simulink model "sampleModel7293_pp_1_1"  (R2018a)
settings: Solver=VariableStepAuto  StartTime=0.0  StopTime=10.0  RelTol=1e-3
undefined symbols (not defined in the file): DiscIntNeverNeededParam
libraries: simulink x367
(part 3 of 9)

== system sampleModel7293_pp_1_1/cfblk183 ==
  cfblk1 : Inport
  cfblk10 : Inport  Port=2
  cfblk11 : Inport  Port=3
  Action Port : ActionPort  ActionType=else
  cfblk15 : Delay
  cfblk3 : Delay  ShowEnablePort=on
      settings: InputPortMap=u0,e6
  cfblk4 : DiscreteFilter
  cfblk5 : DiscreteStateSpace  SampleTime=-1
  cfblk6 : DiscreteStateSpace  SampleTime=-1
  cfblk7 : Delay
  cfblk8 : DiscreteStateSpace  SampleTime=-1
  cfblk9 : simulink/Continuous/PID Controller  Controller=PID  TimeDomain=Discrete-time  SampleTime=-1  IntegratorMethod=Forward Euler  FilterMethod=Forward Euler  Form=Parallel  UseFilter=on  ControllerParametersSource=internal  P=1  I=1  D=0  N=100  InitialConditionSource=internal  InitialConditionForIntegrator=0  InitialConditionForFilter=0  ExternalReset=none  LimitOutput=off  UpperSaturationLimit=inf  LowerSaturationLimit=-inf  LinearizeAsGain=off  AntiWindupMode=none  Kb=1  TrackingMode=off  Kt=1  PParamMin=[]  PParamMax=[]  IParamMin=[]  IParamMax=[]  DParamMin=[]  DParamMax=[]  NParamMin=[]  NParamMax=[]  KbParamMin=[]  KbParamMax=[]  KtParamMin=[]  KtParamMax=[]  POutMin=[]  POutMax=[]  IOutMin=[]  IOutMax=[]  DOutMin=[]  DOutMax=[]  NOutMin=[]  NOutMax=[]  KbOutMin=[]  KbOutMax=[]  KtOutMin=[]  KtOutMax=[]  IntegratorOutMin=[]  IntegratorOutMax=[]  FilterOutMin=[]  FilterOutMax=[]  SumOutMin=[]  SumOutMax=[]  SumI1OutMin=[]  SumI1OutMax=[]  SumI2OutMin=[]  SumI2OutMax=[]  SumI3OutMin=[]  SumI3OutMax=[]  SumDOutMin=[]  SumDOutMax=[]  SaturationOutMin=[]  SaturationOutMax=[]  IntegratorContinuousStateAttributes=''  IntegratorStateMustResolveToSignalObject=off  IntegratorRTWStateStorageClass=Auto  FilterContinuousStateAttributes=''  FilterStateMustResolveToSignalObject=off  FilterRTWStateStorageClass=Auto  DifferentiatorICPrevScaledInput=0  DifferentiatorOutMin=[]  DifferentiatorOutMax=[]  FilterDiffOutCoefMin=[]  FilterDiffOutCoefMax=[]  SumDenOutMin=[]  SumDenOutMax=[]  SumNumOutMin=[]  SumNumOutMax=[]  ReciprocalOutMin=[]  ReciprocalOutMax=[]  DivideOutMin=[]  DivideOutMax=[]  TunerSelectOption=Transfer Function Based (PID Tuner App)
  cyemi_{518..526} (9 alike) : DataTypeConversion  OutDataTypeStr=double
  cfblk2 : Outport
  cfblk12 : Outport  Port=2
  cfblk13 : Outport  Port=3
  cfblk14 : Outport  Port=4
  wires:
  cfblk1/1 -> cfblk14/1
  cfblk4/1 -> cfblk12/1
  cfblk7/1 -> cfblk2/1, cyemi_525/1
  cfblk5/1 -> cfblk13/1, cyemi_524/1
  cyemi_518/1 -> cfblk15/1
  cfblk8/1 -> cyemi_518/1
  cyemi_519/1 -> cfblk3/1
  cfblk15/1 -> cyemi_519/1
  cyemi_520/1 -> cfblk3/2
  cfblk10/1 -> cyemi_520/1
  cyemi_521/1 -> cfblk4/1
  cfblk6/1 -> cyemi_521/1
  cyemi_522/1 -> cfblk5/1
  cfblk9/1 -> cyemi_522/1
  cyemi_523/1 -> cfblk6/1
  cfblk11/1 -> cyemi_523/1
  cyemi_524/1 -> cfblk7/1
  cyemi_525/1 -> cfblk8/1
  cyemi_526/1 -> cfblk9/1
  cfblk3/1 -> cyemi_526/1

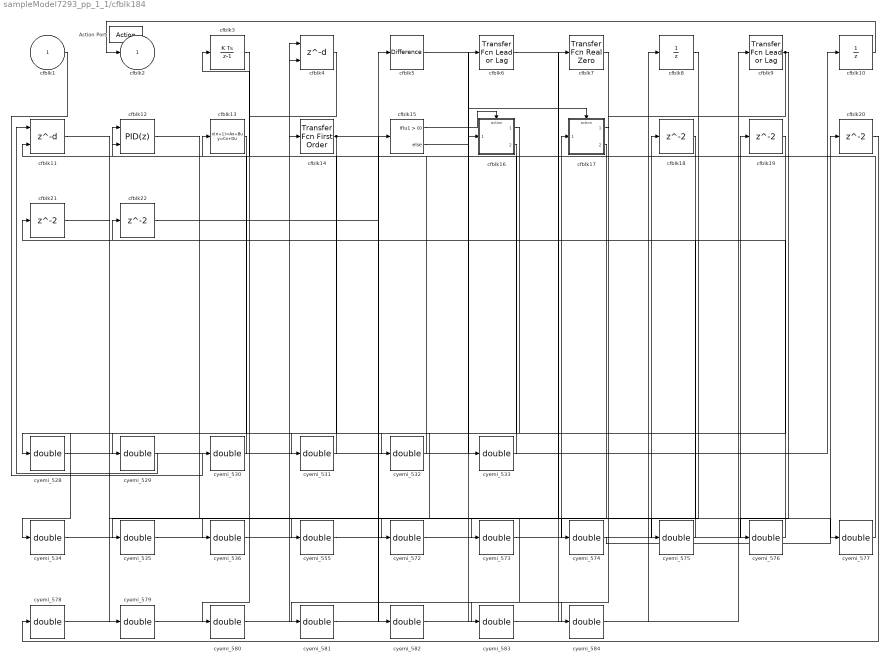
== system sampleModel7293_pp_1_1/cfblk184 ==
  cfblk1 : Inport
  Action Port : ActionPort  ActionType=then
  cfblk10 : UnitDelay  SampleTime=-1
  cfblk11 : Delay  DelayLengthSource=Input port
      settings: InputPortMap=u0,p1
  cfblk12 : simulink/Continuous/PID Controller (2DOF)  Controller=PID  TimeDomain=Discrete-time  SampleTime=-1  IntegratorMethod=Forward Euler  FilterMethod=Forward Euler  Form=Parallel  UseFilter=on  ControllerParametersSource=internal  P=1  I=1  D=0  N=100  b=1  c=1  InitialConditionSource=internal  InitialConditionForIntegrator=0  InitialConditionForFilter=0  ExternalReset=none  LimitOutput=off  UpperSaturationLimit=inf  LowerSaturationLimit=-inf  LinearizeAsGain=off  AntiWindupMode=none  Kb=1  TrackingMode=off  Kt=1  PParamMin=[]  PParamMax=[]  IParamMin=[]  IParamMax=[]  DParamMin=[]  DParamMax=[]  NParamMin=[]  NParamMax=[]  bParamMin=[]  bParamMax=[]  cParamMin=[]  cParamMax=[]  KbParamMin=[]  KbParamMax=[]  KtParamMin=[]  KtParamMax=[]  POutMin=[]  POutMax=[]  IOutMin=[]  IOutMax=[]  DOutMin=[]  DOutMax=[]  NOutMin=[]  NOutMax=[]  bOutMin=[]  bOutMax=[]  cOutMin=[]  cOutMax=[]  KbOutMin=[]  KbOutMax=[]  KtOutMin=[]  KtOutMax=[]  IntegratorOutMin=[]  IntegratorOutMax=[]  FilterOutMin=[]  FilterOutMax=[]  SumOutMin=[]  SumOutMax=[]  Sum1OutMin=[]  Sum1OutMax=[]  Sum2OutMin=[]  Sum2OutMax=[]  Sum3OutMin=[]  Sum3OutMax=[]  SumI1OutMin=[]  SumI1OutMax=[]  SumI2OutMin=[]  SumI2OutMax=[]  SumI3OutMin=[]  SumI3OutMax=[]  SumDOutMin=[]  SumDOutMax=[]  SaturationOutMin=[]  SaturationOutMax=[]  IntegratorContinuousStateAttributes=''  IntegratorStateMustResolveToSignalObject=off  IntegratorRTWStateStorageClass=Auto  FilterContinuousStateAttributes=''  FilterStateMustResolveToSignalObject=off  FilterRTWStateStorageClass=Auto  DifferentiatorICPrevScaledInput=0  DifferentiatorOutMin=[]  DifferentiatorOutMax=[]  FilterDiffOutCoefMin=[]  FilterDiffOutCoefMax=[]  SumDenOutMin=[]  SumDenOutMax=[]  SumNumOutMin=[]  SumNumOutMax=[]  ReciprocalOutMin=[]  ReciprocalOutMax=[]  DivideOutMin=[]  DivideOutMax=[]  TunerSelectOption=Transfer Function Based (PID Tuner App)
  cfblk13 : DiscreteStateSpace  SampleTime=-1
  cfblk14 : simulink/Discrete/Transfer Fcn First Order  PoleZ=0.95  ICPrevOutput=0.0  DoSatur=off
      settings: SourceProductName=Simulink
  cfblk15 : If  SampleTime=1
  cfblk16 : Subsystem  TreatAsAtomicUnit=on
  cfblk17 : Subsystem  TreatAsAtomicUnit=on
  cfblk{18..22} (5 alike) : Delay
  cfblk3 : DiscreteIntegrator  SampleTime=-1  OutDataTypeStr=double  ICPrevOutput=DiscIntNeverNeededParam  ICPrevScaledInput=DiscIntNeverNeededParam
  cfblk4 : Delay  DelayLengthSource=Input port
      settings: InputPortMap=u0,p1
  cfblk5 : simulink/Discrete/Difference  ICPrevInput=0.0  OutMin=[]  OutMax=[]  OutDataTypeStr=double  OutputDataTypeScalingMode=double  OutDataType=fixdt(1, 16)  OutScaling=2^-10  DoSatur=off
  cfblk6 : simulink/Discrete/Transfer Fcn Lead or Lag  PoleZ=0.95  ZeroZ=0.75  ICPrevOutput=0.0  ICPrevInput=0.0  DoSatur=off
      settings: SourceProductName=Simulink  SourceProductBaseCode=SL
  cfblk7 : simulink/Discrete/Transfer Fcn Real Zero  ZeroZ=0.75  ICPrevInput=0.0  DoSatur=off
      settings: SourceProductName=Simulink  SourceProductBaseCode=SL
  cfblk8 : UnitDelay  SampleTime=-1
  cfblk9 : simulink/Discrete/Transfer Fcn Lead or Lag  PoleZ=0.95  ZeroZ=0.75  ICPrevOutput=0.0  ICPrevInput=0.0  DoSatur=off
      settings: SourceProductName=Simulink  SourceProductBaseCode=SL
  cyemi_{528..536,555,572..584} (23 alike) : DataTypeConversion  OutDataTypeStr=double
  cfblk2 : Outport
  wires:
  cfblk14/1 -> cyemi_531/1, cyemi_573/1
  cfblk9/1 -> cyemi_532/1, cyemi_576/1
  cfblk10/1 -> cfblk2/1
  cfblk15/1 -> cfblk16/Action
  cfblk15/2 -> cfblk17/Action
  cyemi_528/1 -> cfblk10/1
  cfblk16/1(cfblk2) -> cyemi_528/1
  cyemi_529/1 -> cfblk11/1
  cfblk19/1 -> cyemi_529/1
  cyemi_530/1 -> cfblk11/2
  cfblk1/1 -> cyemi_530/1
  cyemi_531/1 -> cfblk12/1
  cyemi_532/1 -> cfblk12/2
  cyemi_533/1 -> cfblk13/1
  cfblk5/1 -> cyemi_533/1
  cyemi_534/1 -> cfblk14/1
  cfblk13/1 -> cyemi_534/1
  cyemi_535/1 -> cfblk15/1
  cfblk18/1 -> cyemi_535/1
  cyemi_536/1 -> cfblk16/1(cfblk1)
  cfblk4/1 -> cyemi_536/1
  cyemi_555/1 -> cfblk17/1(cfblk1)
  cfblk21/1 -> cyemi_555/1
  cyemi_572/1 -> cfblk18/1
  cfblk16/2(cfblk16) -> cyemi_572/1
  cyemi_573/1 -> cfblk19/1
  cyemi_574/1 -> cfblk20/1
  cfblk12/1 -> cyemi_574/1
  cyemi_575/1 -> cfblk21/1
  cfblk8/1 -> cyemi_575/1
  cyemi_576/1 -> cfblk22/1
  cyemi_577/1 -> cfblk3/1
  cfblk6/1 -> cyemi_577/1
  cyemi_578/1 -> cfblk4/1
  cfblk20/1 -> cyemi_578/1
  cyemi_579/1 -> cfblk4/2
  cfblk11/1 -> cyemi_579/1
  cyemi_580/1 -> cfblk5/1
  cfblk3/1 -> cyemi_580/1
  cyemi_581/1 -> cfblk6/1
  cfblk17/1(cfblk2) -> cyemi_581/1
  cyemi_582/1 -> cfblk7/1
  cfblk22/1 -> cyemi_582/1
  cyemi_583/1 -> cfblk8/1
  cfblk17/2(cfblk15) -> cyemi_583/1
  cyemi_584/1 -> cfblk9/1
  cfblk7/1 -> cyemi_584/1

== system sampleModel7293_pp_1_1/cfblk185 ==
  cfblk1 : Inport
  cfblk12 : Inport  Port=2
  cfblk13 : Inport  Port=3
  cfblk14 : Inport  Port=4
  cfblk15 : Inport  Port=5
  cfblk16 : Inport  Port=6
  Action Port : ActionPort  ActionType=else
  cfblk10 : Delay  DelayLengthSource=Input port
      settings: InputPortMap=u0,p1
  cfblk11 : If  SampleTime=1
  cfblk18 : Subsystem  TreatAsAtomicUnit=on
  cfblk19 : Subsystem  TreatAsAtomicUnit=on
  cfblk20 : Delay
  cfblk3 : simulink/Discrete/Transfer Fcn First Order  PoleZ=0.95  ICPrevOutput=0.0  DoSatur=off
      settings: SourceProductName=Simulink
  cfblk4 : simulink/Continuous/PID Controller (2DOF)  Controller=PID  TimeDomain=Discrete-time  SampleTime=-1  IntegratorMethod=Forward Euler  FilterMethod=Forward Euler  Form=Parallel  UseFilter=on  ControllerParametersSource=internal  P=1  I=1  D=0  N=100  b=1  c=1  InitialConditionSource=internal  InitialConditionForIntegrator=0  InitialConditionForFilter=0  ExternalReset=none  LimitOutput=off  UpperSaturationLimit=inf  LowerSaturationLimit=-inf  LinearizeAsGain=off  AntiWindupMode=none  Kb=1  TrackingMode=off  Kt=1  PParamMin=[]  PParamMax=[]  IParamMin=[]  IParamMax=[]  DParamMin=[]  DParamMax=[]  NParamMin=[]  NParamMax=[]  bParamMin=[]  bParamMax=[]  cParamMin=[]  cParamMax=[]  KbParamMin=[]  KbParamMax=[]  KtParamMin=[]  KtParamMax=[]  POutMin=[]  POutMax=[]  IOutMin=[]  IOutMax=[]  DOutMin=[]  DOutMax=[]  NOutMin=[]  NOutMax=[]  bOutMin=[]  bOutMax=[]  cOutMin=[]  cOutMax=[]  KbOutMin=[]  KbOutMax=[]  KtOutMin=[]  KtOutMax=[]  IntegratorOutMin=[]  IntegratorOutMax=[]  FilterOutMin=[]  FilterOutMax=[]  SumOutMin=[]  SumOutMax=[]  Sum1OutMin=[]  Sum1OutMax=[]  Sum2OutMin=[]  Sum2OutMax=[]  Sum3OutMin=[]  Sum3OutMax=[]  SumI1OutMin=[]  SumI1OutMax=[]  SumI2OutMin=[]  SumI2OutMax=[]  SumI3OutMin=[]  SumI3OutMax=[]  SumDOutMin=[]  SumDOutMax=[]  SaturationOutMin=[]  SaturationOutMax=[]  IntegratorContinuousStateAttributes=''  IntegratorStateMustResolveToSignalObject=off  IntegratorRTWStateStorageClass=Auto  FilterContinuousStateAttributes=''  FilterStateMustResolveToSignalObject=off  FilterRTWStateStorageClass=Auto  DifferentiatorICPrevScaledInput=0  DifferentiatorOutMin=[]  DifferentiatorOutMax=[]  FilterDiffOutCoefMin=[]  FilterDiffOutCoefMax=[]  SumDenOutMin=[]  SumDenOutMax=[]  SumNumOutMin=[]  SumNumOutMax=[]  ReciprocalOutMin=[]  ReciprocalOutMax=[]  DivideOutMin=[]  DivideOutMax=[]  TunerSelectOption=Transfer Function Based (PID Tuner App)
  cfblk5 : simulink/Discrete/Tapped Delay  vinit=0.0  samptime=-1  NumDelays=1  DelayOrder=Oldest  includeCurrent=off
  cfblk6 : simulink/Discrete/Transfer Fcn Lead or Lag  PoleZ=0.95  ZeroZ=0.75  ICPrevOutput=0.0  ICPrevInput=0.0  DoSatur=off
      settings: SourceProductName=Simulink  SourceProductBaseCode=SL
  cfblk7 : simulink/Continuous/PID Controller (2DOF)  Controller=PID  TimeDomain=Discrete-time  SampleTime=-1  IntegratorMethod=Forward Euler  FilterMethod=Forward Euler  Form=Parallel  UseFilter=on  ControllerParametersSource=internal  P=1  I=1  D=0  N=100  b=1  c=1  InitialConditionSource=internal  InitialConditionForIntegrator=0  InitialConditionForFilter=0  ExternalReset=none  LimitOutput=off  UpperSaturationLimit=inf  LowerSaturationLimit=-inf  LinearizeAsGain=off  AntiWindupMode=none  Kb=1  TrackingMode=off  Kt=1  PParamMin=[]  PParamMax=[]  IParamMin=[]  IParamMax=[]  DParamMin=[]  DParamMax=[]  NParamMin=[]  NParamMax=[]  bParamMin=[]  bParamMax=[]  cParamMin=[]  cParamMax=[]  KbParamMin=[]  KbParamMax=[]  KtParamMin=[]  KtParamMax=[]  POutMin=[]  POutMax=[]  IOutMin=[]  IOutMax=[]  DOutMin=[]  DOutMax=[]  NOutMin=[]  NOutMax=[]  bOutMin=[]  bOutMax=[]  cOutMin=[]  cOutMax=[]  KbOutMin=[]  KbOutMax=[]  KtOutMin=[]  KtOutMax=[]  IntegratorOutMin=[]  IntegratorOutMax=[]  FilterOutMin=[]  FilterOutMax=[]  SumOutMin=[]  SumOutMax=[]  Sum1OutMin=[]  Sum1OutMax=[]  Sum2OutMin=[]  Sum2OutMax=[]  Sum3OutMin=[]  Sum3OutMax=[]  SumI1OutMin=[]  SumI1OutMax=[]  SumI2OutMin=[]  SumI2OutMax=[]  SumI3OutMin=[]  SumI3OutMax=[]  SumDOutMin=[]  SumDOutMax=[]  SaturationOutMin=[]  SaturationOutMax=[]  IntegratorContinuousStateAttributes=''  IntegratorStateMustResolveToSignalObject=off  IntegratorRTWStateStorageClass=Auto  FilterContinuousStateAttributes=''  FilterStateMustResolveToSignalObject=off  FilterRTWStateStorageClass=Auto  DifferentiatorICPrevScaledInput=0  DifferentiatorOutMin=[]  DifferentiatorOutMax=[]  FilterDiffOutCoefMin=[]  FilterDiffOutCoefMax=[]  SumDenOutMin=[]  SumDenOutMax=[]  SumNumOutMin=[]  SumNumOutMax=[]  ReciprocalOutMin=[]  ReciprocalOutMax=[]  DivideOutMin=[]  DivideOutMax=[]  TunerSelectOption=Transfer Function Based (PID Tuner App)
  cfblk8 : DiscreteFilter
  cfblk9 : DiscreteTransferFcn
  cyemi_{591..595,607,616..625} (16 alike) : DataTypeConversion  OutDataTypeStr=double
  cfblk2 : Outport
  cfblk17 : Outport  Port=2
  wires:
  cfblk7/1 -> cfblk17/1
  cfblk6/1 -> cfblk2/1
  cfblk11/1 -> cfblk18/Action
  cfblk11/2 -> cfblk19/Action
  cyemi_591/1 -> cfblk10/1
  cfblk19/1(cfblk2) -> cyemi_591/1
  cyemi_592/1 -> cfblk10/2
  cfblk4/1 -> cyemi_592/1
  cyemi_593/1 -> cfblk11/1
  cfblk5/1 -> cyemi_593/1
  cyemi_594/1 -> cfblk18/1(cfblk1)
  cfblk9/1 -> cyemi_594/1
  cyemi_595/1 -> cfblk18/2(cfblk11)
  cfblk12/1 -> cyemi_595/1
  cyemi_607/1 -> cfblk19/1(cfblk1)
  cfblk18/2(cfblk12) -> cyemi_607/1
  cyemi_616/1 -> cfblk20/1
  cfblk18/1(cfblk2) -> cyemi_616/1
  cyemi_617/1 -> cfblk3/1
  cfblk20/1 -> cyemi_617/1
  cyemi_618/1 -> cfblk4/1
  cfblk16/1 -> cyemi_618/1
  cyemi_619/1 -> cfblk4/2
  cfblk13/1 -> cyemi_619/1
  cyemi_620/1 -> cfblk5/1
  cfblk8/1 -> cyemi_620/1
  cyemi_621/1 -> cfblk6/1
  cfblk15/1 -> cyemi_621/1
  cyemi_622/1 -> cfblk7/1
  cfblk1/1 -> cyemi_622/1
  cyemi_623/1 -> cfblk7/2
  cfblk10/1 -> cyemi_623/1
  cyemi_624/1 -> cfblk8/1
  cfblk14/1 -> cyemi_624/1
  cyemi_625/1 -> cfblk9/1
  cfblk3/1 -> cyemi_625/1

== system sampleModel7293_pp_1_1/cfblk186 ==
  cfblk1 : Inport
  cfblk5 : Inport  Port=2
  cfblk6 : Inport  Port=3
  cfblk7 : Inport  Port=4
  Action Port : ActionPort  ActionType=then
  cfblk3 : Delay  ShowEnablePort=on
      settings: InputPortMap=u0,e6
  cfblk4 : simulink/Discrete/Difference  ICPrevInput=0.0  OutMin=[]  OutMax=[]  OutDataTypeStr=double  OutputDataTypeScalingMode=double  OutDataType=fixdt(1, 16)  OutScaling=2^-10  DoSatur=off
  cyemi_630 : DataTypeConversion  OutDataTypeStr=double
  cyemi_631 : DataTypeConversion  OutDataTypeStr=double
  cyemi_632 : DataTypeConversion  OutDataTypeStr=double
  cfblk2 : Outport
  cfblk8 : Outport  Port=2
  wires:
  cfblk5/1 -> cfblk2/1
  cfblk7/1 -> cfblk8/1
  cyemi_630/1 -> cfblk3/1
  cfblk1/1 -> cyemi_630/1
  cyemi_631/1 -> cfblk3/2
  cfblk4/1 -> cyemi_631/1
  cyemi_632/1 -> cfblk4/1
  cfblk6/1 -> cyemi_632/1

== system sampleModel7293_pp_1_1/cfblk187 ==
  cfblk1 : Inport
  cfblk8 : Inport  Port=2
  cfblk9 : Inport  Port=3
  Action Port : ActionPort  ActionType=else
  cfblk11 : Subsystem  TreatAsAtomicUnit=on
  cfblk12 : Subsystem  TreatAsAtomicUnit=on
  cfblk13 : Delay
  cfblk14 : Delay
  cfblk15 : Delay
  cfblk3 : simulink/Continuous/PID Controller (2DOF)  Controller=PID  TimeDomain=Discrete-time  SampleTime=-1  IntegratorMethod=Forward Euler  FilterMethod=Forward Euler  Form=Parallel  UseFilter=on  ControllerParametersSource=internal  P=1  I=1  D=0  N=100  b=1  c=1  InitialConditionSource=internal  InitialConditionForIntegrator=0  InitialConditionForFilter=0  ExternalReset=none  LimitOutput=off  UpperSaturationLimit=inf  LowerSaturationLimit=-inf  LinearizeAsGain=off  AntiWindupMode=none  Kb=1  TrackingMode=off  Kt=1  PParamMin=[]  PParamMax=[]  IParamMin=[]  IParamMax=[]  DParamMin=[]  DParamMax=[]  NParamMin=[]  NParamMax=[]  bParamMin=[]  bParamMax=[]  cParamMin=[]  cParamMax=[]  KbParamMin=[]  KbParamMax=[]  KtParamMin=[]  KtParamMax=[]  POutMin=[]  POutMax=[]  IOutMin=[]  IOutMax=[]  DOutMin=[]  DOutMax=[]  NOutMin=[]  NOutMax=[]  bOutMin=[]  bOutMax=[]  cOutMin=[]  cOutMax=[]  KbOutMin=[]  KbOutMax=[]  KtOutMin=[]  KtOutMax=[]  IntegratorOutMin=[]  IntegratorOutMax=[]  FilterOutMin=[]  FilterOutMax=[]  SumOutMin=[]  SumOutMax=[]  Sum1OutMin=[]  Sum1OutMax=[]  Sum2OutMin=[]  Sum2OutMax=[]  Sum3OutMin=[]  Sum3OutMax=[]  SumI1OutMin=[]  SumI1OutMax=[]  SumI2OutMin=[]  SumI2OutMax=[]  SumI3OutMin=[]  SumI3OutMax=[]  SumDOutMin=[]  SumDOutMax=[]  SaturationOutMin=[]  SaturationOutMax=[]  IntegratorContinuousStateAttributes=''  IntegratorStateMustResolveToSignalObject=off  IntegratorRTWStateStorageClass=Auto  FilterContinuousStateAttributes=''  FilterStateMustResolveToSignalObject=off  FilterRTWStateStorageClass=Auto  DifferentiatorICPrevScaledInput=0  DifferentiatorOutMin=[]  DifferentiatorOutMax=[]  FilterDiffOutCoefMin=[]  FilterDiffOutCoefMax=[]  SumDenOutMin=[]  SumDenOutMax=[]  SumNumOutMin=[]  SumNumOutMax=[]  ReciprocalOutMin=[]  ReciprocalOutMax=[]  DivideOutMin=[]  DivideOutMax=[]  TunerSelectOption=Transfer Function Based (PID Tuner App)
  cfblk4 : simulink/Discrete/Tapped Delay  vinit=0.0  samptime=-1  NumDelays=1  DelayOrder=Oldest  includeCurrent=off
  cfblk5 : simulink/Continuous/PID Controller (2DOF)  Controller=PID  TimeDomain=Discrete-time  SampleTime=-1  IntegratorMethod=Forward Euler  FilterMethod=Forward Euler  Form=Parallel  UseFilter=on  ControllerParametersSource=internal  P=1  I=1  D=0  N=100  b=1  c=1  InitialConditionSource=internal  InitialConditionForIntegrator=0  InitialConditionForFilter=0  ExternalReset=none  LimitOutput=off  UpperSaturationLimit=inf  LowerSaturationLimit=-inf  LinearizeAsGain=off  AntiWindupMode=none  Kb=1  TrackingMode=off  Kt=1  PParamMin=[]  PParamMax=[]  IParamMin=[]  IParamMax=[]  DParamMin=[]  DParamMax=[]  NParamMin=[]  NParamMax=[]  bParamMin=[]  bParamMax=[]  cParamMin=[]  cParamMax=[]  KbParamMin=[]  KbParamMax=[]  KtParamMin=[]  KtParamMax=[]  POutMin=[]  POutMax=[]  IOutMin=[]  IOutMax=[]  DOutMin=[]  DOutMax=[]  NOutMin=[]  NOutMax=[]  bOutMin=[]  bOutMax=[]  cOutMin=[]  cOutMax=[]  KbOutMin=[]  KbOutMax=[]  KtOutMin=[]  KtOutMax=[]  IntegratorOutMin=[]  IntegratorOutMax=[]  FilterOutMin=[]  FilterOutMax=[]  SumOutMin=[]  SumOutMax=[]  Sum1OutMin=[]  Sum1OutMax=[]  Sum2OutMin=[]  Sum2OutMax=[]  Sum3OutMin=[]  Sum3OutMax=[]  SumI1OutMin=[]  SumI1OutMax=[]  SumI2OutMin=[]  SumI2OutMax=[]  SumI3OutMin=[]  SumI3OutMax=[]  SumDOutMin=[]  SumDOutMax=[]  SaturationOutMin=[]  SaturationOutMax=[]  IntegratorContinuousStateAttributes=''  IntegratorStateMustResolveToSignalObject=off  IntegratorRTWStateStorageClass=Auto  FilterContinuousStateAttributes=''  FilterStateMustResolveToSignalObject=off  FilterRTWStateStorageClass=Auto  DifferentiatorICPrevScaledInput=0  DifferentiatorOutMin=[]  DifferentiatorOutMax=[]  FilterDiffOutCoefMin=[]  FilterDiffOutCoefMax=[]  SumDenOutMin=[]  SumDenOutMax=[]  SumNumOutMin=[]  SumNumOutMax=[]  ReciprocalOutMin=[]  ReciprocalOutMax=[]  DivideOutMin=[]  DivideOutMax=[]  TunerSelectOption=Transfer Function Based (PID Tuner App)
  cfblk6 : DiscreteFilter
  cfblk7 : If  SampleTime=1
  cyemi_{636..638,651..653,660..669} (16 alike) : DataTypeConversion  OutDataTypeStr=double
  cfblk2 : Outport
  cfblk10 : Outport  Port=2
  wires:
  cfblk3/1 -> cfblk10/1
  cfblk9/1 -> cyemi_638/1, cyemi_669/1
  cfblk6/1 -> cfblk2/1, cyemi_637/1, cyemi_666/1
  cfblk12/2(cfblk10) -> cyemi_660/1, cyemi_664/1
  cfblk4/1 -> cyemi_661/1, cyemi_662/1
  cfblk7/1 -> cfblk11/Action
  cfblk7/2 -> cfblk12/Action
  cyemi_636/1 -> cfblk11/1(cfblk1)
  cfblk8/1 -> cyemi_636/1
  cyemi_637/1 -> cfblk11/2(cfblk13)
  cyemi_638/1 -> cfblk11/3(cfblk14)
  cyemi_651/1 -> cfblk12/1(cfblk1)
  cfblk5/1 -> cyemi_651/1
  cyemi_652/1 -> cfblk12/2(cfblk8)
  cfblk14/1 -> cyemi_652/1
  cyemi_653/1 -> cfblk12/3(cfblk9)
  cfblk15/1 -> cyemi_653/1
  cyemi_660/1 -> cfblk13/1
  cyemi_661/1 -> cfblk14/1
  cyemi_662/1 -> cfblk15/1
  cyemi_663/1 -> cfblk3/1
  cfblk12/1(cfblk2) -> cyemi_663/1
  cyemi_664/1 -> cfblk3/2
  cyemi_665/1 -> cfblk4/1
  cfblk11/1(cfblk2) -> cyemi_665/1
  cyemi_666/1 -> cfblk5/1
  cyemi_667/1 -> cfblk5/2
  cfblk13/1 -> cyemi_667/1
  cyemi_668/1 -> cfblk6/1
  cfblk1/1 -> cyemi_668/1
  cyemi_669/1 -> cfblk7/1

== system sampleModel7293_pp_1_1/cfblk188 ==
  cfblk1 : Inport
  cfblk9 : Inport  Port=2
  cfblk10 : Inport  Port=3
  cfblk11 : Inport  Port=4
  Action Port : ActionPort  ActionType=then
  cfblk3 : DiscreteTransferFcn
  cfblk4 : DiscreteFir
  cfblk5 : DiscreteZeroPole  Poles=[0 0.5]  Gain=1  SampleTime=-1
  cfblk6 : simulink/Discrete/Transfer Fcn First Order  PoleZ=0.95  ICPrevOutput=0.0  DoSatur=off
      settings: SourceProductName=Simulink
  cfblk7 : UnitDelay  SampleTime=-1
  cfblk8 : DiscreteIntegrator  SampleTime=-1  OutDataTypeStr=double  ICPrevOutput=DiscIntNeverNeededParam  ICPrevScaledInput=DiscIntNeverNeededParam
  cyemi_{674..679} (6 alike) : DataTypeConversion  OutDataTypeStr=double
  cfblk2 : Outport
  cfblk12 : Outport  Port=2
  wires:
  cfblk7/1 -> cfblk12/1
  cfblk4/1 -> cfblk2/1
  cyemi_674/1 -> cfblk3/1
  cfblk1/1 -> cyemi_674/1
  cyemi_675/1 -> cfblk4/1
  cfblk5/1 -> cyemi_675/1
  cyemi_676/1 -> cfblk5/1
  cfblk6/1 -> cyemi_676/1
  cyemi_677/1 -> cfblk6/1
  cfblk8/1 -> cyemi_677/1
  cyemi_678/1 -> cfblk7/1
  cfblk11/1 -> cyemi_678/1
  cyemi_679/1 -> cfblk8/1
  cfblk3/1 -> cyemi_679/1

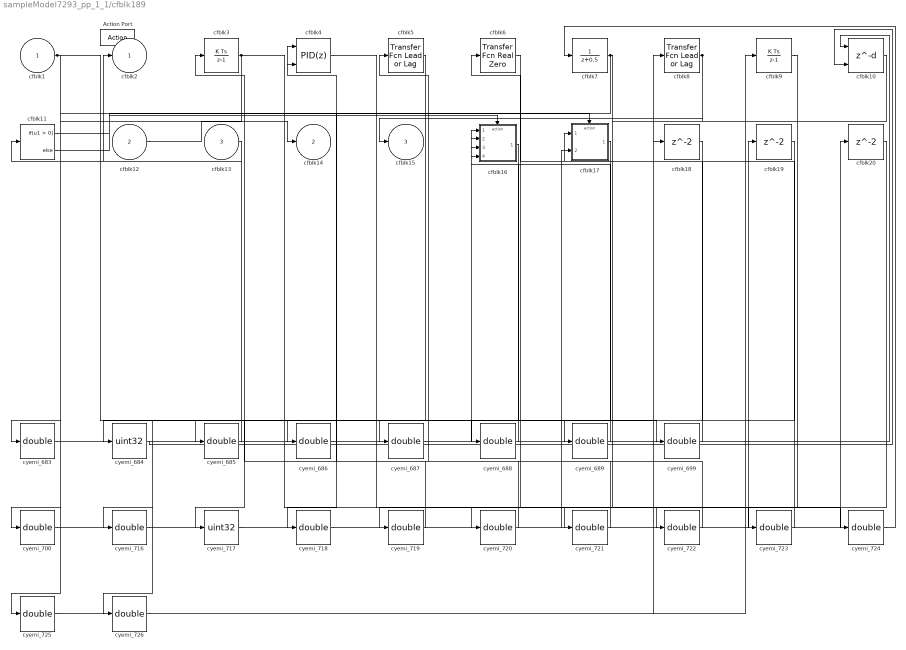
== system sampleModel7293_pp_1_1/cfblk189 ==
  cfblk1 : Inport
  cfblk12 : Inport  Port=2
  cfblk13 : Inport  Port=3
  Action Port : ActionPort  ActionType=else
  cfblk10 : Delay  DelayLengthSource=Input port
      settings: InputPortMap=u0,p1
  cfblk11 : If  SampleTime=1
  cfblk16 : Subsystem  TreatAsAtomicUnit=on
  cfblk17 : Subsystem  TreatAsAtomicUnit=on
  cfblk18 : Delay
  cfblk19 : Delay
  cfblk20 : Delay
  cfblk3 : DiscreteIntegrator  SampleTime=-1  OutDataTypeStr=double  ICPrevOutput=DiscIntNeverNeededParam  ICPrevScaledInput=DiscIntNeverNeededParam
  cfblk4 : simulink/Continuous/PID Controller (2DOF)  Controller=PID  TimeDomain=Discrete-time  SampleTime=-1  IntegratorMethod=Forward Euler  FilterMethod=Forward Euler  Form=Parallel  UseFilter=on  ControllerParametersSource=internal  P=1  I=1  D=0  N=100  b=1  c=1  InitialConditionSource=internal  InitialConditionForIntegrator=0  InitialConditionForFilter=0  ExternalReset=none  LimitOutput=off  UpperSaturationLimit=inf  LowerSaturationLimit=-inf  LinearizeAsGain=off  AntiWindupMode=none  Kb=1  TrackingMode=off  Kt=1  PParamMin=[]  PParamMax=[]  IParamMin=[]  IParamMax=[]  DParamMin=[]  DParamMax=[]  NParamMin=[]  NParamMax=[]  bParamMin=[]  bParamMax=[]  cParamMin=[]  cParamMax=[]  KbParamMin=[]  KbParamMax=[]  KtParamMin=[]  KtParamMax=[]  POutMin=[]  POutMax=[]  IOutMin=[]  IOutMax=[]  DOutMin=[]  DOutMax=[]  NOutMin=[]  NOutMax=[]  bOutMin=[]  bOutMax=[]  cOutMin=[]  cOutMax=[]  KbOutMin=[]  KbOutMax=[]  KtOutMin=[]  KtOutMax=[]  IntegratorOutMin=[]  IntegratorOutMax=[]  FilterOutMin=[]  FilterOutMax=[]  SumOutMin=[]  SumOutMax=[]  Sum1OutMin=[]  Sum1OutMax=[]  Sum2OutMin=[]  Sum2OutMax=[]  Sum3OutMin=[]  Sum3OutMax=[]  SumI1OutMin=[]  SumI1OutMax=[]  SumI2OutMin=[]  SumI2OutMax=[]  SumI3OutMin=[]  SumI3OutMax=[]  SumDOutMin=[]  SumDOutMax=[]  SaturationOutMin=[]  SaturationOutMax=[]  IntegratorContinuousStateAttributes=''  IntegratorStateMustResolveToSignalObject=off  IntegratorRTWStateStorageClass=Auto  FilterContinuousStateAttributes=''  FilterStateMustResolveToSignalObject=off  FilterRTWStateStorageClass=Auto  DifferentiatorICPrevScaledInput=0  DifferentiatorOutMin=[]  DifferentiatorOutMax=[]  FilterDiffOutCoefMin=[]  FilterDiffOutCoefMax=[]  SumDenOutMin=[]  SumDenOutMax=[]  SumNumOutMin=[]  SumNumOutMax=[]  ReciprocalOutMin=[]  ReciprocalOutMax=[]  DivideOutMin=[]  DivideOutMax=[]  TunerSelectOption=Transfer Function Based (PID Tuner App)
  cfblk5 : simulink/Discrete/Transfer Fcn Lead or Lag  PoleZ=0.95  ZeroZ=0.75  ICPrevOutput=0.0  ICPrevInput=0.0  DoSatur=off
      settings: SourceProductName=Simulink  SourceProductBaseCode=SL
  cfblk6 : simulink/Discrete/Transfer Fcn Real Zero  ZeroZ=0.75  ICPrevInput=0.0  DoSatur=off
      settings: SourceProductName=Simulink  SourceProductBaseCode=SL
  cfblk7 : DiscreteTransferFcn
  cfblk8 : simulink/Discrete/Transfer Fcn Lead or Lag  PoleZ=0.95  ZeroZ=0.75  ICPrevOutput=0.0  ICPrevInput=0.0  DoSatur=off
      settings: SourceProductName=Simulink  SourceProductBaseCode=SL
  cfblk9 : DiscreteIntegrator  SampleTime=-1  OutDataTypeStr=double  ICPrevOutput=DiscIntNeverNeededParam  ICPrevScaledInput=DiscIntNeverNeededParam
  cyemi_{683,685..689,699..700,716,718..726} (18 alike) : DataTypeConversion  OutDataTypeStr=double
  cyemi_684 : DataTypeConversion  OutDataTypeStr=uint32
  cyemi_717 : DataTypeConversion  OutDataTypeStr=uint32
  cfblk2 : Outport
  cfblk14 : Outport  Port=2
  cfblk15 : Outport  Port=3
  wires:
  cfblk1/1 -> cyemi_683/1, cyemi_687/1
  cfblk12/1 -> cfblk14/1
  cfblk7/1 -> cyemi_688/1, cyemi_718/1, cyemi_721/1, cyemi_725/1
  cfblk3/1 -> cyemi_699/1, cyemi_700/1, cyemi_724/1
  cfblk8/1 -> cfblk15/1, cyemi_689/1
  cfblk13/1 -> cfblk2/1
  cfblk11/1 -> cfblk16/Action
  cfblk11/2 -> cfblk17/Action
  cyemi_683/1 -> cfblk10/1
  cyemi_684/1 -> cfblk10/2
  cfblk19/1 -> cyemi_684/1
  cyemi_685/1 -> cfblk11/1
  cfblk10/1 -> cyemi_685/1
  cyemi_686/1 -> cfblk16/1(cfblk1)
  cfblk18/1 -> cyemi_686/1
  cyemi_687/1 -> cfblk16/2(cfblk11)
  cyemi_688/1 -> cfblk16/3(cfblk12)
  cyemi_689/1 -> cfblk16/4(cfblk13)
  cyemi_699/1 -> cfblk17/1(cfblk1)
  cyemi_700/1 -> cfblk17/2(cfblk15)
  cyemi_716/1 -> cfblk18/1
  cfblk5/1 -> cyemi_716/1
  cyemi_717/1 -> cfblk19/1
  cfblk17/1(cfblk2) -> cyemi_717/1
  cyemi_718/1 -> cfblk20/1
  cyemi_719/1 -> cfblk3/1
  cfblk20/1 -> cyemi_719/1
  cyemi_720/1 -> cfblk4/1
  cfblk6/1 -> cyemi_720/1
  cyemi_721/1 -> cfblk4/2
  cyemi_722/1 -> cfblk5/1
  cfblk4/1 -> cyemi_722/1
  cyemi_723/1 -> cfblk6/1
  cfblk9/1 -> cyemi_723/1
  cyemi_724/1 -> cfblk7/1
  cyemi_725/1 -> cfblk8/1
  cyemi_726/1 -> cfblk9/1
  cfblk16/1(cfblk2) -> cyemi_726/1

== system sampleModel7293_pp_1_1/cfblk190 ==
  cfblk1 : Inport
  Action Port : ActionPort  ActionType=then
  cfblk10 : Subsystem  TreatAsAtomicUnit=on
  cfblk11 : Delay
  cfblk12 : Delay
  cfblk13 : Delay
  cfblk3 : simulink/Discrete/Transfer Fcn Lead or Lag  PoleZ=0.95  ZeroZ=0.75  ICPrevOutput=0.0  ICPrevInput=0.0  DoSatur=off
      settings: SourceProductName=Simulink  SourceProductBaseCode=SL
  cfblk4 : UnitDelay  SampleTime=-1
  cfblk5 : simulink/Discrete/Transfer Fcn Real Zero  ZeroZ=0.75  ICPrevInput=0.0  DoSatur=off
      settings: SourceProductName=Simulink  SourceProductBaseCode=SL
  cfblk6 : If  SampleTime=1
  cfblk9 : Subsystem  TreatAsAtomicUnit=on
  cyemi_{729..730,749..756} (10 alike) : DataTypeConversion  OutDataTypeStr=double
  cfblk2 : Outport
  cfblk7 : Outport  Port=2
  cfblk8 : Outport  Port=3
  wires:
  cfblk9/1(cfblk2) -> cfblk2/1, cyemi_754/1
  cfblk10/2(cfblk15) -> cfblk7/1, cyemi_753/1
  cfblk4/1 -> cfblk8/1, cyemi_751/1
  cfblk6/1 -> cfblk9/Action
  cfblk6/2 -> cfblk10/Action
  cyemi_729/1 -> cfblk10/1(cfblk1)
  cfblk11/1 -> cyemi_729/1
  cyemi_730/1 -> cfblk10/2(cfblk14)
  cfblk1/1 -> cyemi_730/1
  cyemi_749/1 -> cfblk11/1
  cfblk3/1 -> cyemi_749/1
  cyemi_750/1 -> cfblk12/1
  cfblk10/1(cfblk2) -> cyemi_750/1
  cyemi_751/1 -> cfblk13/1
  cyemi_752/1 -> cfblk3/1
  cfblk5/1 -> cyemi_752/1
  cyemi_753/1 -> cfblk4/1
  cyemi_754/1 -> cfblk5/1
  cyemi_755/1 -> cfblk6/1
  cfblk12/1 -> cyemi_755/1
  cyemi_756/1 -> cfblk9/1(cfblk1)
  cfblk13/1 -> cyemi_756/1

== system sampleModel7293_pp_1_1/cfblk191 ==
  cfblk1 : Inport
  cfblk8 : Inport  Port=2
  Action Port : ActionPort  ActionType=else
  cfblk10 : Delay
  cfblk3 : DiscreteFir
  cfblk4 : simulink/Continuous/PID Controller (2DOF)  Controller=PID  TimeDomain=Discrete-time  SampleTime=-1  IntegratorMethod=Forward Euler  FilterMethod=Forward Euler  Form=Parallel  UseFilter=on  ControllerParametersSource=internal  P=1  I=1  D=0  N=100  b=1  c=1  InitialConditionSource=internal  InitialConditionForIntegrator=0  InitialConditionForFilter=0  ExternalReset=none  LimitOutput=off  UpperSaturationLimit=inf  LowerSaturationLimit=-inf  LinearizeAsGain=off  AntiWindupMode=none  Kb=1  TrackingMode=off  Kt=1  PParamMin=[]  PParamMax=[]  IParamMin=[]  IParamMax=[]  DParamMin=[]  DParamMax=[]  NParamMin=[]  NParamMax=[]  bParamMin=[]  bParamMax=[]  cParamMin=[]  cParamMax=[]  KbParamMin=[]  KbParamMax=[]  KtParamMin=[]  KtParamMax=[]  POutMin=[]  POutMax=[]  IOutMin=[]  IOutMax=[]  DOutMin=[]  DOutMax=[]  NOutMin=[]  NOutMax=[]  bOutMin=[]  bOutMax=[]  cOutMin=[]  cOutMax=[]  KbOutMin=[]  KbOutMax=[]  KtOutMin=[]  KtOutMax=[]  IntegratorOutMin=[]  IntegratorOutMax=[]  FilterOutMin=[]  FilterOutMax=[]  SumOutMin=[]  SumOutMax=[]  Sum1OutMin=[]  Sum1OutMax=[]  Sum2OutMin=[]  Sum2OutMax=[]  Sum3OutMin=[]  Sum3OutMax=[]  SumI1OutMin=[]  SumI1OutMax=[]  SumI2OutMin=[]  SumI2OutMax=[]  SumI3OutMin=[]  SumI3OutMax=[]  SumDOutMin=[]  SumDOutMax=[]  SaturationOutMin=[]  SaturationOutMax=[]  IntegratorContinuousStateAttributes=''  IntegratorStateMustResolveToSignalObject=off  IntegratorRTWStateStorageClass=Auto  FilterContinuousStateAttributes=''  FilterStateMustResolveToSignalObject=off  FilterRTWStateStorageClass=Auto  DifferentiatorICPrevScaledInput=0  DifferentiatorOutMin=[]  DifferentiatorOutMax=[]  FilterDiffOutCoefMin=[]  FilterDiffOutCoefMax=[]  SumDenOutMin=[]  SumDenOutMax=[]  SumNumOutMin=[]  SumNumOutMax=[]  ReciprocalOutMin=[]  ReciprocalOutMax=[]  DivideOutMin=[]  DivideOutMax=[]  TunerSelectOption=Transfer Function Based (PID Tuner App)
  cfblk5 : simulink/Discrete/Transfer Fcn Real Zero  ZeroZ=0.75  ICPrevInput=0.0  DoSatur=off
      settings: SourceProductName=Simulink  SourceProductBaseCode=SL
  cfblk6 : Delay  DelayLengthSource=Input port
      settings: InputPortMap=u0,p1
  cfblk7 : DiscreteStateSpace  SampleTime=-1
  cfblk9 : Delay
  cyemi_{772..780} (9 alike) : DataTypeConversion  OutDataTypeStr=double
  cfblk2 : Outport
  wires:
  cfblk8/1 -> cfblk2/1
  cfblk6/1 -> cyemi_773/1, cyemi_780/1
  cyemi_772/1 -> cfblk10/1
  cfblk3/1 -> cyemi_772/1
  cyemi_773/1 -> cfblk3/1
  cyemi_774/1 -> cfblk4/1
  cfblk7/1 -> cyemi_774/1
  cyemi_775/1 -> cfblk4/2
  cfblk9/1 -> cyemi_775/1
  cyemi_776/1 -> cfblk5/1
  cfblk1/1 -> cyemi_776/1
  cyemi_777/1 -> cfblk6/1
  cfblk4/1 -> cyemi_777/1
  cyemi_778/1 -> cfblk6/2
  cfblk10/1 -> cyemi_778/1
  cyemi_779/1 -> cfblk7/1
  cfblk5/1 -> cyemi_779/1
  cyemi_780/1 -> cfblk9/1

== system sampleModel7293_pp_1_1/cfblk192 ==
  cfblk1 : Inport
  cfblk9 : Inport  Port=2
  cfblk10 : Inport  Port=3
  Action Port : ActionPort  ActionType=then
  cfblk3 : DiscreteTransferFcn
  cfblk4 : simulink/Discrete/Tapped Delay  vinit=0.0  samptime=-1  NumDelays=1  DelayOrder=Oldest  includeCurrent=off
  cfblk5 : DiscreteFir
  cfblk6 : Delay  DelayLengthSource=Input port
      settings: InputPortMap=u0,p1
  cfblk7 : simulink/Discrete/Difference  ICPrevInput=0.0  OutMin=[]  OutMax=[]  OutDataTypeStr=double  OutputDataTypeScalingMode=double  OutDataType=fixdt(1, 16)  OutScaling=2^-10  DoSatur=off
  cfblk8 : DiscreteTransferFcn
  cyemi_{784..790} (7 alike) : DataTypeConversion  OutDataTypeStr=double
  cfblk2 : Outport
  cfblk11 : Outport  Port=2
  wires:
  cfblk10/1 -> cfblk2/1
  cfblk5/1 -> cfblk11/1
  cyemi_784/1 -> cfblk3/1
  cfblk6/1 -> cyemi_784/1
  cyemi_785/1 -> cfblk4/1
  cfblk8/1 -> cyemi_785/1
  cyemi_786/1 -> cfblk5/1
  cfblk7/1 -> cyemi_786/1
  cyemi_787/1 -> cfblk6/1
  cfblk1/1 -> cyemi_787/1
  cyemi_788/1 -> cfblk6/2
  cfblk4/1 -> cyemi_788/1
  cyemi_789/1 -> cfblk7/1
  cfblk3/1 -> cyemi_789/1
  cyemi_790/1 -> cfblk8/1
  cfblk9/1 -> cyemi_790/1

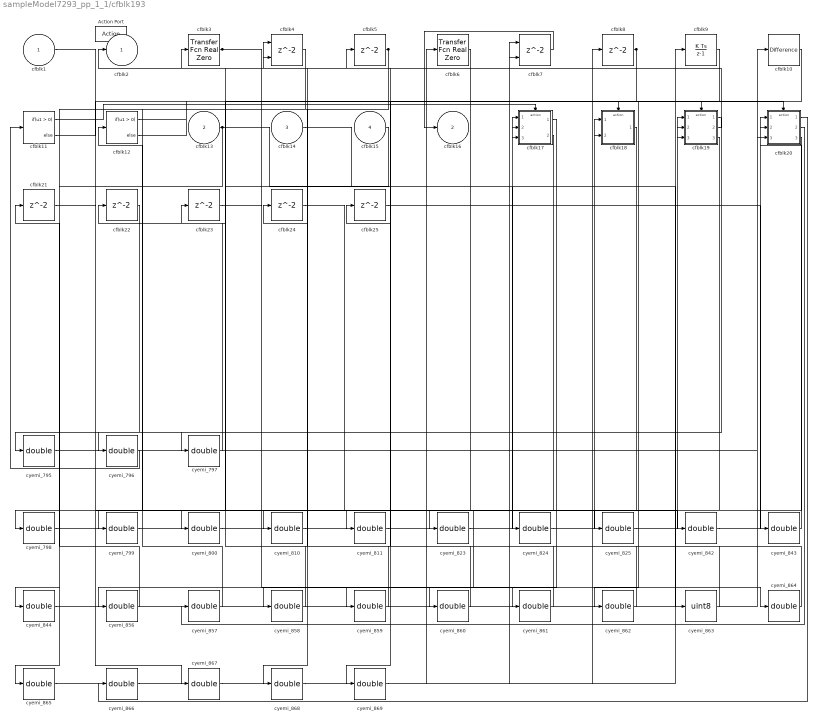
== system sampleModel7293_pp_1_1/cfblk193 ==
  cfblk1 : Inport
  cfblk13 : Inport  Port=2
  cfblk14 : Inport  Port=3
  cfblk15 : Inport  Port=4
  Action Port : ActionPort  ActionType=else
  cfblk10 : simulink/Discrete/Difference  ICPrevInput=0.0  OutMin=[]  OutMax=[]  OutDataTypeStr=double  OutputDataTypeScalingMode=double  OutDataType=fixdt(1, 16)  OutScaling=2^-10  DoSatur=off
  cfblk11 : If  SampleTime=1
  cfblk12 : If  SampleTime=1
  cfblk17 : Subsystem  TreatAsAtomicUnit=on
  cfblk18 : Subsystem  TreatAsAtomicUnit=on
  cfblk19 : Subsystem  TreatAsAtomicUnit=on
  cfblk20 : Subsystem  TreatAsAtomicUnit=on
  cfblk{5,8,21..25} (7 alike) : Delay
  cfblk3 : simulink/Discrete/Transfer Fcn Real Zero  ZeroZ=0.75  ICPrevInput=0.0  DoSatur=off
      settings: SourceProductName=Simulink  SourceProductBaseCode=SL
  cfblk4 : Delay  ShowEnablePort=on
      settings: InputPortMap=u0,e6
  cfblk6 : simulink/Discrete/Transfer Fcn Real Zero  ZeroZ=0.75  ICPrevInput=0.0  DoSatur=off
      settings: SourceProductName=Simulink  SourceProductBaseCode=SL
  cfblk7 : Delay  ShowEnablePort=on
      settings: InputPortMap=u0,e6
  cfblk9 : DiscreteIntegrator  SampleTime=-1  OutDataTypeStr=double  ICPrevOutput=DiscIntNeverNeededParam  ICPrevScaledInput=DiscIntNeverNeededParam
  cyemi_{795..800,810..811,823..825,842..844,856..862,864..869} (27 alike) : DataTypeConversion  OutDataTypeStr=double
  cyemi_863 : DataTypeConversion  OutDataTypeStr=uint8
  cfblk2 : Outport
  cfblk16 : Outport  Port=2
  wires:
  cfblk7/1 -> cfblk16/1
  cfblk5/1 -> cyemi_799/1, cyemi_868/1
  cfblk19/2(cfblk15) -> cfblk2/1
  cfblk8/1 -> cyemi_800/1, cyemi_823/1
  cfblk3/1 -> cyemi_811/1, cyemi_864/1
  cfblk13/1 -> cyemi_824/1, cyemi_844/1
  cfblk11/1 -> cfblk17/Action
  cfblk11/2 -> cfblk18/Action
  cfblk12/1 -> cfblk19/Action
  cfblk12/2 -> cfblk20/Action
  cyemi_795/1 -> cfblk10/1
  cfblk19/1(cfblk2) -> cyemi_795/1
  cyemi_796/1 -> cfblk11/1
  cfblk22/1 -> cyemi_796/1
  cyemi_797/1 -> cfblk12/1
  cfblk15/1 -> cyemi_797/1
  cyemi_798/1 -> cfblk17/1(cfblk1)
  cfblk4/1 -> cyemi_798/1
  cyemi_799/1 -> cfblk17/2(cfblk12)
  cyemi_800/1 -> cfblk17/3(cfblk13)
  cyemi_810/1 -> cfblk18/1(cfblk1)
  cfblk19/3(cfblk16) -> cyemi_810/1
  cyemi_811/1 -> cfblk18/2(cfblk11)
  cyemi_823/1 -> cfblk19/1(cfblk1)
  cyemi_824/1 -> cfblk19/2(cfblk13)
  cyemi_825/1 -> cfblk19/3(cfblk14)
  cfblk24/1 -> cyemi_825/1
  cyemi_842/1 -> cfblk20/1(cfblk1)
  cfblk21/1 -> cyemi_842/1
  cyemi_843/1 -> cfblk20/2(cfblk13)
  cfblk25/1 -> cyemi_843/1
  cyemi_844/1 -> cfblk20/3(cfblk14)
  cyemi_856/1 -> cfblk21/1
  cfblk17/1(cfblk2) -> cyemi_856/1
  cyemi_857/1 -> cfblk22/1
  cfblk20/2(cfblk15) -> cyemi_857/1
  cyemi_858/1 -> cfblk23/1
  cfblk6/1 -> cyemi_858/1
  cyemi_859/1 -> cfblk24/1
  cfblk20/3(cfblk16) -> cyemi_859/1
  cyemi_860/1 -> cfblk25/1
  cfblk17/2(cfblk14) -> cyemi_860/1
  cyemi_861/1 -> cfblk3/1
  cfblk23/1 -> cyemi_861/1
  cyemi_862/1 -> cfblk4/1
  cfblk9/1 -> cyemi_862/1
  cyemi_863/1 -> cfblk4/2
  cfblk14/1 -> cyemi_863/1
  cyemi_864/1 -> cfblk5/1
  cyemi_865/1 -> cfblk6/1
  cfblk18/1(cfblk2) -> cyemi_865/1
  cyemi_866/1 -> cfblk7/1
  cfblk20/1(cfblk2) -> cyemi_866/1
  cyemi_867/1 -> cfblk7/2
  cfblk1/1 -> cyemi_867/1
  cyemi_868/1 -> cfblk8/1
  cyemi_869/1 -> cfblk9/1
  cfblk10/1 -> cyemi_869/1

== system sampleModel7293_pp_1_1/cfblk194 ==
  cfblk1 : Inport
  Action Port : ActionPort  ActionType=then
  cfblk3 : Delay
  cfblk4 : simulink/Continuous/PID Controller  Controller=PID  TimeDomain=Discrete-time  SampleTime=-1  IntegratorMethod=Forward Euler  FilterMethod=Forward Euler  Form=Parallel  UseFilter=on  ControllerParametersSource=internal  P=1  I=1  D=0  N=100  InitialConditionSource=internal  InitialConditionForIntegrator=0  InitialConditionForFilter=0  ExternalReset=none  LimitOutput=off  UpperSaturationLimit=inf  LowerSaturationLimit=-inf  LinearizeAsGain=off  AntiWindupMode=none  Kb=1  TrackingMode=off  Kt=1  PParamMin=[]  PParamMax=[]  IParamMin=[]  IParamMax=[]  DParamMin=[]  DParamMax=[]  NParamMin=[]  NParamMax=[]  KbParamMin=[]  KbParamMax=[]  KtParamMin=[]  KtParamMax=[]  POutMin=[]  POutMax=[]  IOutMin=[]  IOutMax=[]  DOutMin=[]  DOutMax=[]  NOutMin=[]  NOutMax=[]  KbOutMin=[]  KbOutMax=[]  KtOutMin=[]  KtOutMax=[]  IntegratorOutMin=[]  IntegratorOutMax=[]  FilterOutMin=[]  FilterOutMax=[]  SumOutMin=[]  SumOutMax=[]  SumI1OutMin=[]  SumI1OutMax=[]  SumI2OutMin=[]  SumI2OutMax=[]  SumI3OutMin=[]  SumI3OutMax=[]  SumDOutMin=[]  SumDOutMax=[]  SaturationOutMin=[]  SaturationOutMax=[]  IntegratorContinuousStateAttributes=''  IntegratorStateMustResolveToSignalObject=off  IntegratorRTWStateStorageClass=Auto  FilterContinuousStateAttributes=''  FilterStateMustResolveToSignalObject=off  FilterRTWStateStorageClass=Auto  DifferentiatorICPrevScaledInput=0  DifferentiatorOutMin=[]  DifferentiatorOutMax=[]  FilterDiffOutCoefMin=[]  FilterDiffOutCoefMax=[]  SumDenOutMin=[]  SumDenOutMax=[]  SumNumOutMin=[]  SumNumOutMax=[]  ReciprocalOutMin=[]  ReciprocalOutMax=[]  DivideOutMin=[]  DivideOutMax=[]  TunerSelectOption=Transfer Function Based (PID Tuner App)
  cfblk5 : UnitDelay  SampleTime=-1
  cfblk6 : DiscreteTransferFcn
  cfblk7 : Delay  ShowEnablePort=on
      settings: InputPortMap=u0,e6
  cfblk8 : Delay
  cyemi_{871..877} (7 alike) : DataTypeConversion  OutDataTypeStr=double
  cfblk2 : Outport
  wires:
  cfblk4/1 -> cfblk2/1
  cfblk6/1 -> cyemi_876/1, cyemi_877/1
  cyemi_871/1 -> cfblk3/1
  cfblk8/1 -> cyemi_871/1
  cyemi_872/1 -> cfblk4/1
  cfblk7/1 -> cyemi_872/1
  cyemi_873/1 -> cfblk5/1
  cfblk1/1 -> cyemi_873/1
  cyemi_874/1 -> cfblk6/1
  cfblk3/1 -> cyemi_874/1
  cyemi_875/1 -> cfblk7/1
  cfblk5/1 -> cyemi_875/1
  cyemi_876/1 -> cfblk7/2
  cyemi_877/1 -> cfblk8/1

== system sampleModel7293_pp_1_1/cfblk195 ==
  cfblk1 : Inport
  cfblk7 : Inport  Port=2
  Action Port : ActionPort  ActionType=else
  cfblk{10..13} (4 alike) : Delay
  cfblk3 : Delay  ShowEnablePort=on
      settings: InputPortMap=u0,e6
  cfblk4 : simulink/Discrete/Difference  ICPrevInput=0.0  OutMin=[]  OutMax=[]  OutDataTypeStr=double  OutputDataTypeScalingMode=double  OutDataType=fixdt(1, 16)  OutScaling=2^-10  DoSatur=off
  cfblk5 : simulink/Discrete/Transfer Fcn Lead or Lag  PoleZ=0.95  ZeroZ=0.75  ICPrevOutput=0.0  ICPrevInput=0.0  DoSatur=off
      settings: SourceProductName=Simulink  SourceProductBaseCode=SL
  cfblk6 : If  SampleTime=1
  cfblk8 : Subsystem  TreatAsAtomicUnit=on
  cfblk9 : Subsystem  TreatAsAtomicUnit=on
  cyemi_{880..891,903..906} (16 alike) : DataTypeConversion  OutDataTypeStr=double
  cfblk2 : Outport
  wires:
  cfblk3/1 -> cyemi_883/1, cyemi_887/1
  cfblk5/1 -> cfblk2/1
  cfblk8/1(cfblk2) -> cyemi_880/1, cyemi_882/1, cyemi_886/1
  cfblk9/3(cfblk15) -> cyemi_885/1, cyemi_891/1
  cfblk6/1 -> cfblk8/Action
  cfblk6/2 -> cfblk9/Action
  cyemi_880/1 -> cfblk10/1
  cyemi_881/1 -> cfblk11/1
  cfblk4/1 -> cyemi_881/1
  cyemi_882/1 -> cfblk12/1
  cyemi_883/1 -> cfblk13/1
  cyemi_884/1 -> cfblk3/1
  cfblk7/1 -> cyemi_884/1
  cyemi_885/1 -> cfblk3/2
  cyemi_886/1 -> cfblk4/1
  cyemi_887/1 -> cfblk5/1
  cyemi_888/1 -> cfblk6/1
  cfblk11/1 -> cyemi_888/1
  cyemi_889/1 -> cfblk8/1(cfblk1)
  cfblk9/1(cfblk2) -> cyemi_889/1
  cyemi_890/1 -> cfblk8/2(cfblk11)
  cfblk9/2(cfblk14) -> cyemi_890/1
  cyemi_891/1 -> cfblk8/3(cfblk12)
  cyemi_903/1 -> cfblk9/1(cfblk1)
  cfblk10/1 -> cyemi_903/1
  cyemi_904/1 -> cfblk9/2(cfblk11)
  cfblk1/1 -> cyemi_904/1
  cyemi_905/1 -> cfblk9/3(cfblk12)
  cfblk13/1 -> cyemi_905/1
  cyemi_906/1 -> cfblk9/4(cfblk13)
  cfblk12/1 -> cyemi_906/1

== system sampleModel7293_pp_1_1/cfblk196 ==
  cfblk1 : Inport
  cfblk9 : Inport  Port=2
  cfblk10 : Inport  Port=3
  Action Port : ActionPort  ActionType=then
  cfblk11 : Subsystem  TreatAsAtomicUnit=on
  cfblk12 : Subsystem  TreatAsAtomicUnit=on
  cfblk13 : Delay
  cfblk14 : Delay
  cfblk3 : simulink/Continuous/PID Controller  Controller=PID  TimeDomain=Discrete-time  SampleTime=-1  IntegratorMethod=Forward Euler  FilterMethod=Forward Euler  Form=Parallel  UseFilter=on  ControllerParametersSource=internal  P=1  I=1  D=0  N=100  InitialConditionSource=internal  InitialConditionForIntegrator=0  InitialConditionForFilter=0  ExternalReset=none  LimitOutput=off  UpperSaturationLimit=inf  LowerSaturationLimit=-inf  LinearizeAsGain=off  AntiWindupMode=none  Kb=1  TrackingMode=off  Kt=1  PParamMin=[]  PParamMax=[]  IParamMin=[]  IParamMax=[]  DParamMin=[]  DParamMax=[]  NParamMin=[]  NParamMax=[]  KbParamMin=[]  KbParamMax=[]  KtParamMin=[]  KtParamMax=[]  POutMin=[]  POutMax=[]  IOutMin=[]  IOutMax=[]  DOutMin=[]  DOutMax=[]  NOutMin=[]  NOutMax=[]  KbOutMin=[]  KbOutMax=[]  KtOutMin=[]  KtOutMax=[]  IntegratorOutMin=[]  IntegratorOutMax=[]  FilterOutMin=[]  FilterOutMax=[]  SumOutMin=[]  SumOutMax=[]  SumI1OutMin=[]  SumI1OutMax=[]  SumI2OutMin=[]  SumI2OutMax=[]  SumI3OutMin=[]  SumI3OutMax=[]  SumDOutMin=[]  SumDOutMax=[]  SaturationOutMin=[]  SaturationOutMax=[]  IntegratorContinuousStateAttributes=''  IntegratorStateMustResolveToSignalObject=off  IntegratorRTWStateStorageClass=Auto  FilterContinuousStateAttributes=''  FilterStateMustResolveToSignalObject=off  FilterRTWStateStorageClass=Auto  DifferentiatorICPrevScaledInput=0  DifferentiatorOutMin=[]  DifferentiatorOutMax=[]  FilterDiffOutCoefMin=[]  FilterDiffOutCoefMax=[]  SumDenOutMin=[]  SumDenOutMax=[]  SumNumOutMin=[]  SumNumOutMax=[]  ReciprocalOutMin=[]  ReciprocalOutMax=[]  DivideOutMin=[]  DivideOutMax=[]  TunerSelectOption=Transfer Function Based (PID Tuner App)
  cfblk4 : simulink/Discrete/Transfer Fcn Lead or Lag  PoleZ=0.95  ZeroZ=0.75  ICPrevOutput=0.0  ICPrevInput=0.0  DoSatur=off
      settings: SourceProductName=Simulink  SourceProductBaseCode=SL
  cfblk5 : Delay  ShowEnablePort=on
      settings: InputPortMap=u0,e6
  cfblk6 : DiscreteStateSpace  SampleTime=-1
  cfblk7 : DiscreteIntegrator  SampleTime=-1  OutDataTypeStr=double  ICPrevOutput=DiscIntNeverNeededParam  ICPrevScaledInput=DiscIntNeverNeededParam
  cfblk8 : If  SampleTime=1
  cyemi_{919..921,929,940..948} (13 alike) : DataTypeConversion  OutDataTypeStr=double
  cfblk2 : Outport
  wires:
  cfblk12/1(cfblk2) -> cfblk2/1
  cfblk8/1 -> cfblk11/Action
  cfblk8/2 -> cfblk12/Action
  cyemi_919/1 -> cfblk11/1(cfblk1)
  cfblk14/1 -> cyemi_919/1
  cyemi_920/1 -> cfblk11/2(cfblk10)
  cfblk1/1 -> cyemi_920/1, cyemi_921/1
  cyemi_921/1 -> cfblk11/3(cfblk11)
  cyemi_929/1 -> cfblk12/1(cfblk1)
  cfblk4/1 -> cyemi_929/1
  cyemi_940/1 -> cfblk13/1
  cfblk5/1 -> cyemi_940/1
  cyemi_941/1 -> cfblk14/1
  cfblk7/1 -> cyemi_941/1
  cyemi_942/1 -> cfblk3/1
  cfblk10/1 -> cyemi_942/1
  cyemi_943/1 -> cfblk4/1
  cfblk3/1 -> cyemi_943/1
  cyemi_944/1 -> cfblk5/1
  cfblk9/1 -> cyemi_944/1
  cyemi_945/1 -> cfblk5/2
  cfblk11/1(cfblk2) -> cyemi_945/1
  cyemi_946/1 -> cfblk6/1
  cfblk12/2(cfblk12) -> cyemi_946/1
  cyemi_947/1 -> cfblk7/1
  cfblk6/1 -> cyemi_947/1
  cyemi_948/1 -> cfblk8/1
  cfblk13/1 -> cyemi_948/1

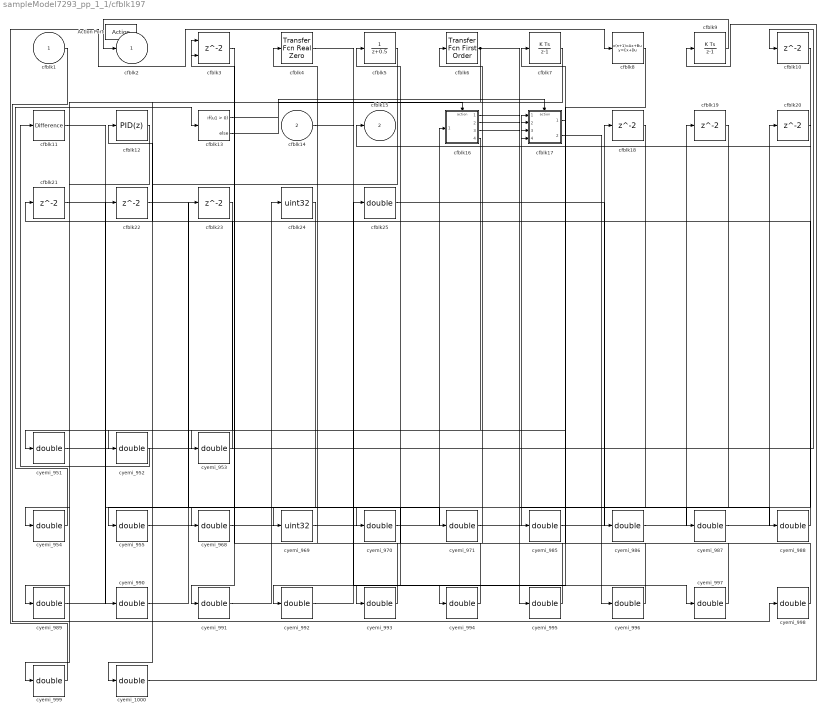
== system sampleModel7293_pp_1_1/cfblk197 ==
  cfblk1 : Inport
  cfblk14 : Inport  Port=2
  Action Port : ActionPort  ActionType=else
  cfblk{10,18..23} (7 alike) : Delay
  cfblk11 : simulink/Discrete/Difference  ICPrevInput=0.0  OutMin=[]  OutMax=[]  OutDataTypeStr=double  OutputDataTypeScalingMode=double  OutDataType=fixdt(1, 16)  OutScaling=2^-10  DoSatur=off
  cfblk12 : simulink/Continuous/PID Controller  Controller=PID  TimeDomain=Discrete-time  SampleTime=-1  IntegratorMethod=Forward Euler  FilterMethod=Forward Euler  Form=Parallel  UseFilter=on  ControllerParametersSource=internal  P=1  I=1  D=0  N=100  InitialConditionSource=internal  InitialConditionForIntegrator=0  InitialConditionForFilter=0  ExternalReset=none  LimitOutput=off  UpperSaturationLimit=inf  LowerSaturationLimit=-inf  LinearizeAsGain=off  AntiWindupMode=none  Kb=1  TrackingMode=off  Kt=1  PParamMin=[]  PParamMax=[]  IParamMin=[]  IParamMax=[]  DParamMin=[]  DParamMax=[]  NParamMin=[]  NParamMax=[]  KbParamMin=[]  KbParamMax=[]  KtParamMin=[]  KtParamMax=[]  POutMin=[]  POutMax=[]  IOutMin=[]  IOutMax=[]  DOutMin=[]  DOutMax=[]  NOutMin=[]  NOutMax=[]  KbOutMin=[]  KbOutMax=[]  KtOutMin=[]  KtOutMax=[]  IntegratorOutMin=[]  IntegratorOutMax=[]  FilterOutMin=[]  FilterOutMax=[]  SumOutMin=[]  SumOutMax=[]  SumI1OutMin=[]  SumI1OutMax=[]  SumI2OutMin=[]  SumI2OutMax=[]  SumI3OutMin=[]  SumI3OutMax=[]  SumDOutMin=[]  SumDOutMax=[]  SaturationOutMin=[]  SaturationOutMax=[]  IntegratorContinuousStateAttributes=''  IntegratorStateMustResolveToSignalObject=off  IntegratorRTWStateStorageClass=Auto  FilterContinuousStateAttributes=''  FilterStateMustResolveToSignalObject=off  FilterRTWStateStorageClass=Auto  DifferentiatorICPrevScaledInput=0  DifferentiatorOutMin=[]  DifferentiatorOutMax=[]  FilterDiffOutCoefMin=[]  FilterDiffOutCoefMax=[]  SumDenOutMin=[]  SumDenOutMax=[]  SumNumOutMin=[]  SumNumOutMax=[]  ReciprocalOutMin=[]  ReciprocalOutMax=[]  DivideOutMin=[]  DivideOutMax=[]  TunerSelectOption=Transfer Function Based (PID Tuner App)
  cfblk13 : If  SampleTime=1
  cfblk16 : Subsystem  TreatAsAtomicUnit=on
  cfblk17 : Subsystem  TreatAsAtomicUnit=on
  cfblk24 : DataTypeConversion  OutDataTypeStr=uint32
  cfblk25 : DataTypeConversion  OutDataTypeStr=double
  cfblk3 : Delay  ShowEnablePort=on
      settings: InputPortMap=u0,e6
  cfblk4 : simulink/Discrete/Transfer Fcn Real Zero  ZeroZ=0.75  ICPrevInput=0.0  DoSatur=off
      settings: SourceProductName=Simulink  SourceProductBaseCode=SL
  cfblk5 : DiscreteTransferFcn
  cfblk6 : simulink/Discrete/Transfer Fcn First Order  PoleZ=0.95  ICPrevOutput=0.0  DoSatur=off
      settings: SourceProductName=Simulink
  cfblk7 : DiscreteIntegrator  SampleTime=-1  OutDataTypeStr=double  ICPrevOutput=DiscIntNeverNeededParam  ICPrevScaledInput=DiscIntNeverNeededParam
  cfblk8 : DiscreteStateSpace  SampleTime=-1
  cfblk9 : DiscreteIntegrator  SampleTime=-1  OutDataTypeStr=double  ICPrevOutput=DiscIntNeverNeededParam  ICPrevScaledInput=DiscIntNeverNeededParam
  cyemi_{951..955,968,970..971,985..1000} (24 alike) : DataTypeConversion  OutDataTypeStr=double
  cyemi_969 : DataTypeConversion  OutDataTypeStr=uint32
  cfblk2 : Outport
  cfblk15 : Outport  Port=2
  wires:
  cfblk10/1 -> cfblk15/1
  cfblk9/1 -> cfblk2/1
  cfblk6/1 -> cyemi_987/1, cyemi_999/1
  cfblk13/1 -> cfblk16/Action
  cfblk13/2 -> cfblk17/Action
  cyemi_951/1 -> cfblk10/1
  cfblk17/1(cfblk2) -> cyemi_951/1
  cyemi_952/1 -> cfblk11/1
  cfblk5/1 -> cyemi_952/1
  cyemi_953/1 -> cfblk12/1
  cfblk16/4(cfblk13) -> cyemi_953/1
  cyemi_954/1 -> cfblk13/1
  cfblk23/1 -> cyemi_954/1
  cyemi_955/1 -> cfblk16/1(cfblk1)
  cfblk20/1 -> cyemi_955/1
  cyemi_968/1 -> cfblk17/1(cfblk1)
  cfblk3/1 -> cyemi_968/1
  cyemi_969/1 -> cfblk17/2(cfblk12)
  cfblk24/1 -> cyemi_969/1
  cyemi_970/1 -> cfblk17/3(cfblk13)
  cfblk22/1 -> cyemi_970/1
  cyemi_971/1 -> cfblk17/4(cfblk14)
  cfblk21/1 -> cyemi_971/1
  cyemi_985/1 -> cfblk18/1
  cfblk16/1(cfblk2) -> cyemi_985/1
  cyemi_986/1 -> cfblk19/1
  cfblk25/1 -> cyemi_986/1
  cyemi_987/1 -> cfblk20/1
  cyemi_988/1 -> cfblk21/1
  cfblk16/3(cfblk12) -> cyemi_988/1
  cyemi_989/1 -> cfblk22/1
  cfblk12/1 -> cyemi_989/1
  cyemi_990/1 -> cfblk23/1
  cfblk11/1 -> cyemi_990/1
  cyemi_991/1 -> cfblk24/1
  cfblk19/1 -> cyemi_991/1
  cyemi_992/1 -> cfblk25/1
  cfblk8/1 -> cyemi_992/1
  cyemi_993/1 -> cfblk3/1
  cfblk18/1 -> cyemi_993/1
  cyemi_994/1 -> cfblk3/2
  cfblk14/1 -> cyemi_994/1
  cyemi_995/1 -> cfblk4/1
  cfblk16/2(cfblk11) -> cyemi_995/1
  cyemi_996/1 -> cfblk5/1
  cfblk17/2(cfblk15) -> cyemi_996/1
  cyemi_997/1 -> cfblk6/1
  cfblk4/1 -> cyemi_997/1
  cyemi_998/1 -> cfblk7/1
  cfblk1/1 -> cyemi_998/1
  cyemi_999/1 -> cfblk8/1
  cyemi_1000/1 -> cfblk9/1
  cfblk7/1 -> cyemi_1000/1
